simulink model "autogenExample"  (R2021a)
settings: Solver=FixedStepAuto  StartTime=0.0  StopTime=T_end  FixedStep=T_step  RelTol=1e-3
undefined symbols (not defined in the file): V_i
settings Model: Creator=Nishanth  LastModifiedBy=Nishanth
settings SolverCC: AlgebraicLoopSolver=TrustRegion
settings DataIOCC: ReturnWorkspaceOutputs=off
settings OptimizationCC: DefaultParameterBehavior=Inlined  EnhancedBackFolding=on  PassReuseOutputArgsAs=Individual arguments  ZeroExternalMemoryAtStartup=off  ZeroInternalMemoryAtStartup=off  OptimizeBlockOrder=speed  DifferentSizesBufferReuse=on  OptimizationCustomize=off  EfficientTunableParamExpr=on
settings DebuggingCC: ParameterTunabilityLossMsg=error  SFMachineParentedDataDiag=warning  ArithmeticOperatorsInVariantConditions=warning
settings SFSimCC: SimUseLocalCustomCode=off  MATLABDynamicMemAlloc=off  CustomCodeUndefinedFunction=UseInterfaceOnly
settings RTWCC: SystemTargetFile=ert.tlc  GenCodeOnly=on  TemplateMakefile=ert_default_tmf  RTWUseLocalCustomCode=off
settings CodeAppCC: ForceParamTrailComments=on  IgnoreCustomStorageClasses=off  OperatorAnnotations=on  SimulinkDataObjDesc=on  SFDataObjDesc=on  InsertBlockDesc=on
settings ERTTargetCC: TargetLangStandard=C99 (ISO)  GenerateSampleERTMain=on  InlinedParameterPlacement=NonHierarchical  ERTCustomFileTemplate=example_file_process.tlc

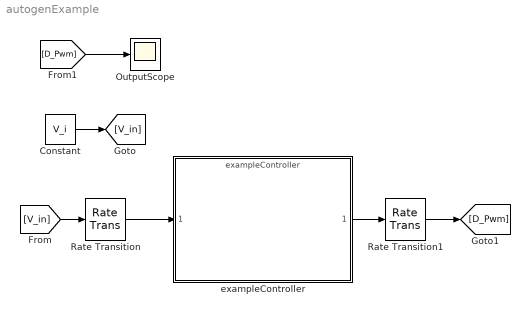
== system autogenExample ==
  Constant : Constant  Value=V_i  SampleTime=50e-3
  OutputScope : Scope
  Rate Transition : RateTransition  OutPortSampleTime=0.0001
  Rate Transition1 : RateTransition  OutPortSampleTime=0.0001
  exampleController : ModelReference  ModelNameDialog=exampleController  SimulationMode=Normal  ModelReferenceVersion=9.0
  wires:
  Constant/1 -> [V_in]
  [D_Pwm] -> OutputScope/1
  Rate Transition/1 -> exampleController/1
  [V_in] -> Rate Transition/1
  exampleController/1 -> Rate Transition1/1
  Rate Transition1/1 -> [D_Pwm]
